simulink model "Designation"  (R2025b)
settings: Solver=VariableStepAuto  StartTime=0.0  StopTime=Tf  RelTol=1e-3
values from neighbouring files (symbols this model uses):
  Kd = (2*zeta*Wn - Pm) / (Km * Pm)    [Designation_matlab.m]
  Ki = 1    [Designation_matlab.m]
  Km = 10.7936 / 10.7132    (= 1.00750476048)    [Designation_mat.m]    (also in Designation_matlab.m = 1301)
  Kp = Wn^2 / (Km * Pm)    (= 0.106517797472)    [Designation_matlab.m]
  Pm = 10.42    [Designation_matlab.m]
settings Model: Creator=ohyus  LastModifiedBy=GILBERT

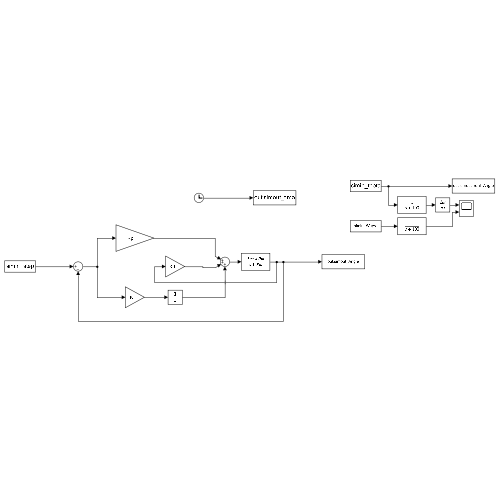
[thumbnail: Simulink's stored preview of the top-level diagram]
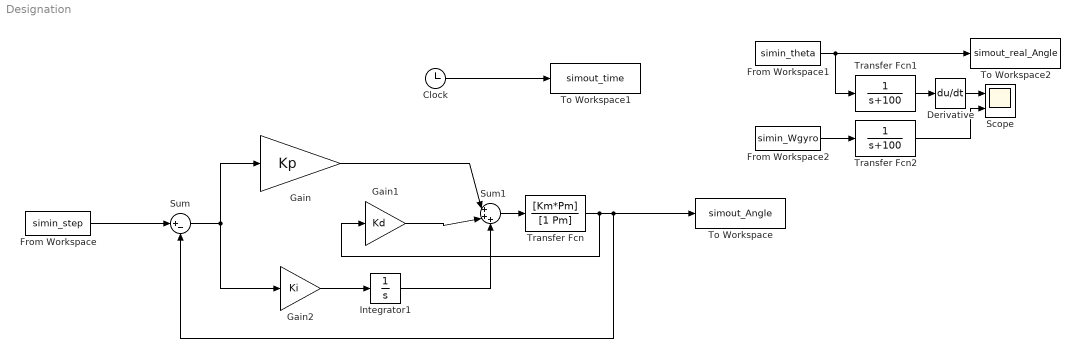
== system Designation ==
  Clock : Clock
  Derivative : Derivative
  From Workspace : FromWorkspace  VariableName=simin_step
  From Workspace1 : FromWorkspace  VariableName=simin_theta
  From Workspace2 : FromWorkspace  VariableName=simin_Wgyro
  Gain : Gain  Gain=Kp
  Gain1 : Gain  Gain=Kd
  Gain2 : Gain  Gain=Ki
  Integrator1 : Integrator
  Scope : Scope  NumInputPorts=2
      settings: ActiveDisplayYMinimum=-4.1118258478011072  ActiveDisplayYMaximum=5.0878341212782114
  Sum : Sum  Inputs=|+-
  Sum1 : Sum  Inputs=|+++
  To Workspace : ToWorkspace  VariableName=simout_Angle  SampleTime=-1
  To Workspace1 : ToWorkspace  VariableName=simout_time  SampleTime=-1
  To Workspace2 : ToWorkspace  VariableName=simout_real_Angle  SampleTime=-1
  Transfer Fcn : TransferFcn  Numerator=[Km*Pm]  Denominator=[1 Pm]
  Transfer Fcn1 : TransferFcn  Denominator=[1 100]
  Transfer Fcn2 : TransferFcn  Denominator=[1 100]
  wires:
  Transfer Fcn/1 -> Gain1/1, To Workspace/1, Sum/2
  Gain/1 -> Sum1/1
  Sum1/1 -> Transfer Fcn/1
  Clock/1 -> To Workspace1/1
  From Workspace/1 -> Sum/1
  From Workspace1/1 -> Transfer Fcn1/1, To Workspace2/1
  Derivative/1 -> Scope/1
  Transfer Fcn1/1 -> Derivative/1
  From Workspace2/1 -> Transfer Fcn2/1
  Transfer Fcn2/1 -> Scope/2
  Gain2/1 -> Integrator1/1
  Integrator1/1 -> Sum1/3
  Sum/1 -> Gain2/1, Gain/1
  Gain1/1 -> Sum1/2
